simulink model "cooSim"  (R2018b)
settings: Solver=VariableStepAuto  StartTime=0.0  StopTime=Time(end)  RelTol=1e-3
values from neighbouring files (symbols this model uses):
  A = [lang.velocity.x(i) lang.velocity.y(i)]'    [DataTreatment.m]    (also in coo.m = [)
  B = [ ... (first row only)    [coo.m]
  C = (R^-1)*A    [DataTreatment.m]    (also in coo.m = [)
  c = rms(sqrt(a.^2+b.^2))    [coo.m]
  D = [ ... (first row only)    [coo.m]
  iz = 4.192e3    (= 4192)    [coo.m]
  Ki = lqi(Gpss,Q,R)    [coo.m]
  lf = cog_x*L    (= 0.70125)    [coo.m]
  lr = (1-cog_x)*L    (= 2.10375)    [coo.m]
  m = m(trimstart:end-trimend,:)    [DataTreatment.m]    (also in coo.m = mean([1684 1774]))
  swaThreshold = 5    [coo.m]
  TH = 9999    [coo.m]
  vxThreshold = 1    [coo.m]
  yawThreshold = 0.1    [coo.m]
undefined symbols (not defined in the file or in its folder): K, Vehicle
libraries: simulink_extras x1
settings Model: Creator=carl  LastModifiedBy=carl

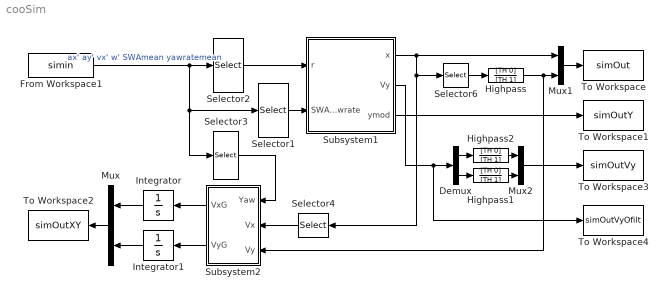
== system cooSim ==
  Demux : Demux  Outputs=2
  From Workspace1 : FromWorkspace  VariableName=simin  SampleTime=0
  Highpass : TransferFcn  Numerator=[TH 0]  Denominator=[TH 1]
  Highpass1 : TransferFcn  Numerator=[TH 0]  Denominator=[TH 1]
  Highpass2 : TransferFcn  Numerator=[TH 0]  Denominator=[TH 1]
  Integrator : Integrator
  Integrator1 : Integrator
  Mux : Mux  Inputs=2
  Mux1 : Mux  Inputs=2
  Mux2 : Mux  Inputs=2
  Selector1 : Selector  InputPortWidth=7  IndexOptions=Index vector (dialog)  Indices=[3,6,7]  OutputSizes=1
  Selector2 : Selector  InputPortWidth=7  IndexOptions=Index vector (dialog)  Indices=[1 2 3 4]  OutputSizes=1
  Selector3 : Selector  InputPortWidth=7  IndexOptions=Index vector (dialog)  Indices=[5]  OutputSizes=1
  Selector4 : Selector  InputPortWidth=3  IndexOptions=Index vector (dialog)  Indices=[1]  OutputSizes=1
  Selector6 : Selector  InputPortWidth=3  IndexOptions=Index vector (dialog)  Indices=[2]  OutputSizes=1
  Subsystem1 : Subsystem
  Subsystem2 : Subsystem
  To Workspace : ToWorkspace  VariableName=simOut  SaveFormat=Timeseries  SampleTime=-1
  To Workspace1 : ToWorkspace  VariableName=simOutY  SaveFormat=Timeseries  SampleTime=-1
  To Workspace2 : ToWorkspace  VariableName=simOutXY  SaveFormat=Timeseries  SampleTime=-1
  To Workspace3 : ToWorkspace  VariableName=simOutVy  SaveFormat=Timeseries  SampleTime=-1
  To Workspace4 : ToWorkspace  VariableName=simOutVyOfilt  SaveFormat=Timeseries  SampleTime=-1
  wires:
  From Workspace1/1 -> Selector1/1, Selector3/1, Selector2/1  "ax' ay' vx' w' SWAmean yawratemean"
  Subsystem1/1(x) -> Selector4/1, Selector6/1, Mux1/1
  Subsystem1/3(ymod) -> To Workspace1/1
  Subsystem2/1(VxG) -> Integrator/1
  Subsystem2/2(VyG) -> Integrator1/1
  Selector3/1 -> Subsystem2/1(Yaw)
  Integrator1/1 -> Mux/2
  Integrator/1 -> Mux/1
  Mux/1 -> To Workspace2/1
  Selector4/1 -> Subsystem2/2(Vx)
  Mux1/1 -> To Workspace/1
  Selector6/1 -> Highpass/1
  Subsystem1/2(Vy) -> To Workspace4/1, Demux/1
  Highpass1/1 -> Mux2/2
  Highpass2/1 -> Mux2/1
  Mux2/1 -> To Workspace3/1
  Demux/1 -> Highpass2/1
  Demux/2 -> Highpass1/1
  Selector2/1 -> Subsystem1/1(r)
  Selector1/1 -> Subsystem1/2(SWA yawrate)
  Highpass/1 -> Subsystem2/3(Vy), Mux1/2

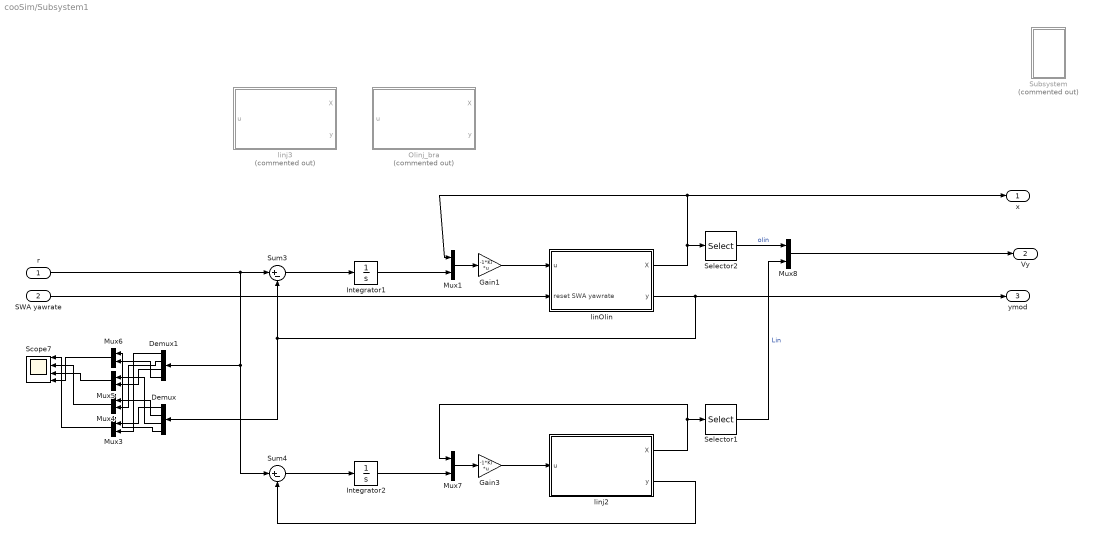
== system cooSim/Subsystem1 ==
  r : Inport
  SWA yawrate : Inport  Port=2
  Demux : Demux
  Demux1 : Demux
  Gain1 : Gain  Gain=-1*Ki  Multiplication=Matrix(K*u) (u vector)
  Gain3 : Gain  Gain=-1*Ki  Multiplication=Matrix(K*u) (u vector)
  Integrator1 : Integrator
  Integrator2 : Integrator
  Mux{1,3..8} (7 alike) : Mux  Inputs=2
  Olinj_bra : Subsystem  Commented=on
  Scope7 : Scope  NumInputPorts=4
  Selector1 : Selector  InputPortWidth=3  IndexOptions=Index vector (dialog)  Indices=2  OutputSizes=1
  Selector2 : Selector  InputPortWidth=3  IndexOptions=Index vector (dialog)  Indices=2  OutputSizes=1
  Subsystem : Subsystem  Commented=on
  Sum3 : Sum  Inputs=|+-
  Sum4 : Sum  Inputs=|+-
  linOlin : Subsystem
  linj2 : Subsystem
  linj3 : Subsystem  Commented=on
  x : Outport
  Vy : Outport  Port=2
  ymod : Outport  Port=3
  wires:
  Sum3/1 -> Integrator1/1
  Gain1/1 -> linOlin/1(u)
  linOlin/2(y) -> Demux/1, Sum3/2, ymod/1
  linOlin/1(X) -> x/1, Mux1/1, Selector2/1
  Mux1/1 -> Gain1/1
  Integrator1/1 -> Mux1/2
  r/1 -> Demux1/1, Sum4/1, Sum3/1
  Selector2/1 -> Mux8/1  "olin"
  Mux3/1 -> Scope7/1
  Mux4/1 -> Scope7/2
  Mux5/1 -> Scope7/3
  Mux6/1 -> Scope7/4
  Demux/1 -> Mux3/1
  Demux1/1 -> Mux3/2
  Demux/2 -> Mux4/1
  Demux1/2 -> Mux4/2
  Demux/3 -> Mux5/1
  Demux1/3 -> Mux5/2
  Demux/4 -> Mux6/1
  Demux1/4 -> Mux6/2
  Selector1/1 -> Mux8/2  "Lin"
  Integrator2/1 -> Mux7/2
  Mux7/1 -> Gain3/1
  linj2/1(X) -> Mux7/1, Selector1/1
  linj2/2(y) -> Sum4/2
  Gain3/1 -> linj2/1(u)
  Sum4/1 -> Integrator2/1
  Mux8/1 -> Vy/1
  SWA yawrate/1 -> linOlin/2(reset SWA yawrate)

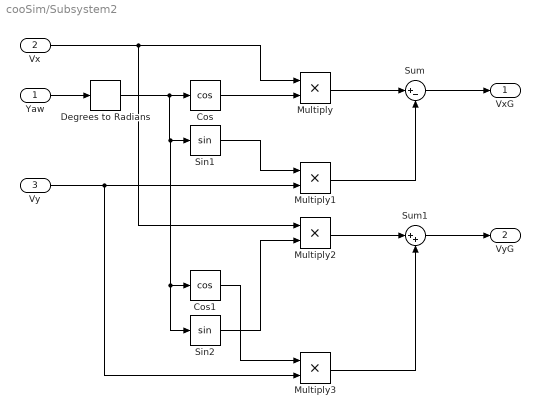
== system cooSim/Subsystem2 ==
  Yaw : Inport
  Vx : Inport  Port=2
  Vy : Inport  Port=3
  Cos : Trigonometry  Operator=cos
  Cos1 : Trigonometry  Operator=cos
  Degrees to Radians : simulink_extras/Transformations/Degrees to Radians
  Multiply{,1..3} (4 alike) : Product
  Sin1 : Trigonometry
  Sin2 : Trigonometry
  Sum : Sum  Inputs=|+-
  Sum1 : Sum  Inputs=|++
  VxG : Outport
  VyG : Outport  Port=2
  wires:
  Multiply/1 -> Sum/1
  Cos/1 -> Multiply/2
  Sin1/1 -> Multiply1/1
  Multiply1/1 -> Sum/2
  Sum/1 -> VxG/1
  Multiply2/1 -> Sum1/1
  Vx/1 -> Multiply2/1, Multiply/1
  Multiply3/1 -> Sum1/2
  Vy/1 -> Multiply1/2, Multiply3/2
  Sum1/1 -> VyG/1
  Sin2/1 -> Multiply2/2
  Cos1/1 -> Multiply3/1
  Yaw/1 -> Degrees to Radians/1
  Degrees to Radians/1 -> Sin2/1, Cos1/1, Sin1/1, Cos/1

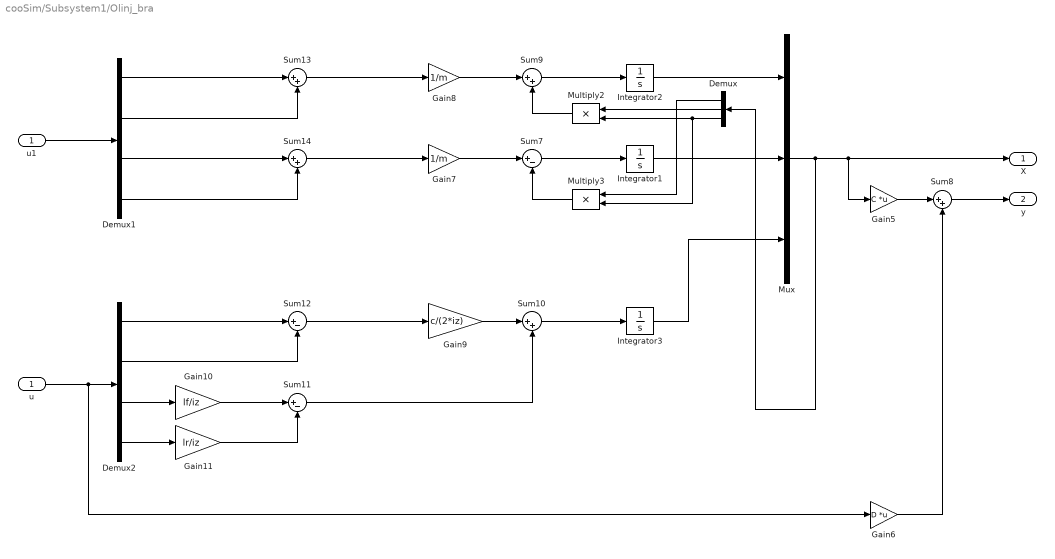
== system cooSim/Subsystem1/Olinj_bra ==
  u : Inport
  Demux : Demux  Outputs=3
  Demux1 : Demux
  Demux2 : Demux
  Gain10 : Gain  Gain=lf/iz
  Gain11 : Gain  Gain=lr/iz
  Gain5 : Gain  Gain=C  Multiplication=Matrix(K*u) (u vector)
  Gain6 : Gain  Gain=D  Multiplication=Matrix(K*u) (u vector)
  Gain7 : Gain  Gain=1/m
  Gain8 : Gain  Gain=1/m
  Gain9 : Gain  Gain=c/(2*iz)
  Integrator1 : Integrator
  Integrator2 : Integrator
  Integrator3 : Integrator
  Multiply2 : Product
  Multiply3 : Product
  Mux : Mux  Inputs=3
  Sum{8..10,13..14} (5 alike) : Sum  Inputs=|++
  Sum11 : Sum  Inputs=|+-
  Sum12 : Sum  Inputs=|+-
  Sum7 : Sum  Inputs=|+-
  u1 : InportShadow
  X : Outport
  y : Outport  Port=2
  wires:
  Gain5/1 -> Sum8/1
  Gain6/1 -> Sum8/2
  Sum8/1 -> y/1
  Gain7/1 -> Sum7/1
  Sum7/1 -> Integrator1/1
  Gain8/1 -> Sum9/1
  Sum9/1 -> Integrator2/1
  Multiply2/1 -> Sum9/2
  Multiply3/1 -> Sum7/2
  Sum10/1 -> Integrator3/1
  Gain9/1 -> Sum10/1
  Gain10/1 -> Sum11/1
  Gain11/1 -> Sum11/2
  u/1 -> Gain6/1, Demux2/1
  Demux2/1 -> Sum12/1
  Demux2/2 -> Sum12/2
  Sum12/1 -> Gain9/1
  Demux2/3 -> Gain10/1
  Demux2/4 -> Gain11/1
  Sum11/1 -> Sum10/2
  u1/1 -> Demux1/1
  Demux1/1 -> Sum13/1
  Demux1/2 -> Sum13/2
  Demux1/3 -> Sum14/1
  Demux1/4 -> Sum14/2
  Sum13/1 -> Gain8/1
  Sum14/1 -> Gain7/1
  Integrator3/1 -> Mux/3
  Integrator1/1 -> Mux/2
  Integrator2/1 -> Mux/1
  Demux/2 -> Multiply2/1
  Demux/1 -> Multiply3/1
  Demux/3 -> Multiply3/2, Multiply2/2
  Mux/1 -> X/1, Gain5/1, Demux/1

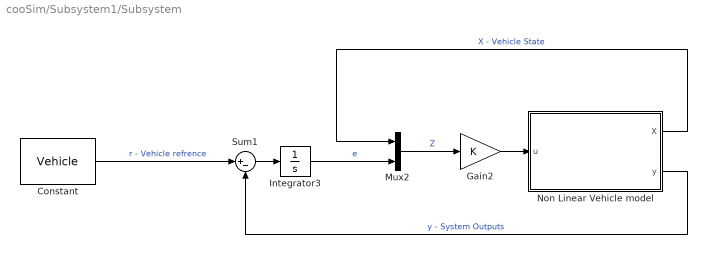
== system cooSim/Subsystem1/Subsystem ==
  Constant : Constant  Value=Vehicle
  Gain2 : Gain  Gain=K
  Integrator3 : Integrator
  Mux2 : Mux  Inputs=2
  Non Linear Vehicle model : Subsystem
  Sum1 : Sum  Inputs=|+-
  wires:
  Gain2/1 -> Non Linear Vehicle model/1(u)
  Sum1/1 -> Integrator3/1
  Constant/1 -> Sum1/1  "r - Vehicle refrence"
  Mux2/1 -> Gain2/1  "Z"
  Non Linear Vehicle model/1(X) -> Mux2/1  "X - Vehicle State"
  Non Linear Vehicle model/2(y) -> Sum1/2  "y - System Outputs"
  Integrator3/1 -> Mux2/2  "e"

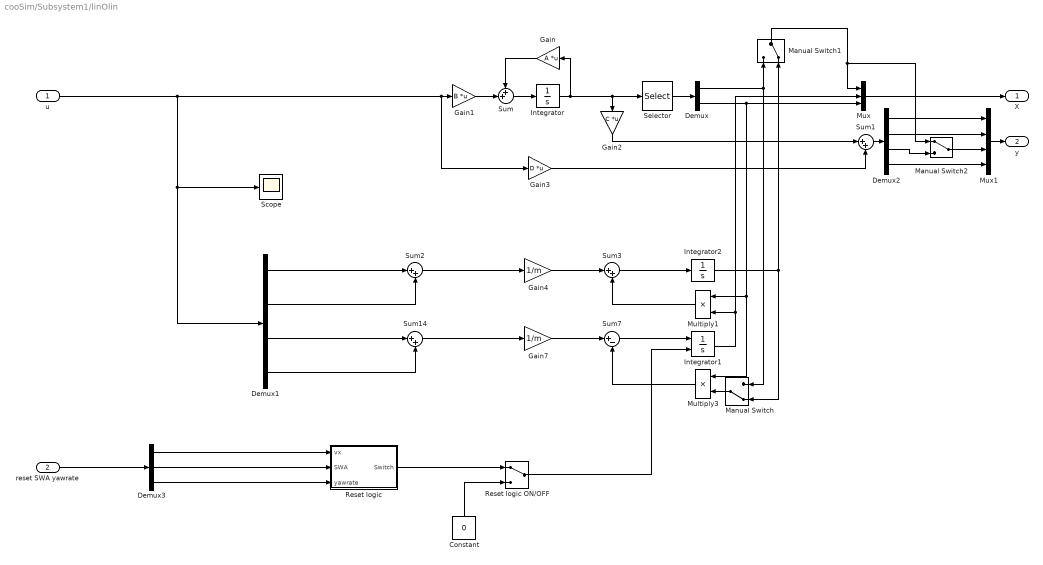
== system cooSim/Subsystem1/linOlin ==
  u : Inport
  reset SWA yawrate : Inport  Port=2
  Constant : Constant  Value=0
  Demux : Demux  Outputs=2
  Demux1 : Demux
  Demux2 : Demux
  Demux3 : Demux  Outputs=3
  Gain : Gain  Gain=A  Multiplication=Matrix(K*u) (u vector)
  Gain1 : Gain  Gain=B  Multiplication=Matrix(K*u) (u vector)
  Gain2 : Gain  Gain=C  Multiplication=Matrix(K*u) (u vector)
  Gain3 : Gain  Gain=D  Multiplication=Matrix(K*u) (u vector)
  Gain4 : Gain  Gain=1/m
  Gain7 : Gain  Gain=1/m
  Integrator : Integrator
  Integrator1 : Integrator  ExternalReset=rising
  Integrator2 : Integrator
  Manual Switch : ManualSwitch  CurrentSetting=0
  Manual Switch1 : ManualSwitch  CurrentSetting=0
  Manual Switch2 : ManualSwitch
  Multiply1 : Product
  Multiply3 : Product
  Mux : Mux  Inputs=3
  Mux1 : Mux
  Reset logic : Subsystem
  Reset logic ON/OFF : ManualSwitch
  Scope : Scope
  Selector : Selector  InputPortWidth=3  IndexOptions=Index vector (dialog)  Indices=[1 3]  OutputSizes=1
  Sum : Sum  Inputs=++|
  Sum{1..3,14} (4 alike) : Sum  Inputs=|++
  Sum7 : Sum  Inputs=|+-
  X : Outport
  y : Outport  Port=2
  wires:
  Sum1/1 -> Demux2/1
  Sum/1 -> Integrator/1
  Integrator/1 -> Gain2/1, Selector/1, Gain/1
  Gain/1 -> Sum/1
  Gain1/1 -> Sum/2
  Gain2/1 -> Sum1/1
  Gain3/1 -> Sum1/2
  Demux/1 -> Manual Switch/1, Manual Switch1/1
  Demux1/4 -> Sum14/2
  Sum7/1 -> Integrator1/1
  Multiply3/1 -> Sum7/2
  Demux1/3 -> Sum14/1
  Sum14/1 -> Gain7/1
  Integrator1/1 -> Multiply1/2, Mux/2
  u/1 -> Gain3/1, Gain1/1, Demux1/1, Scope/1
  Gain7/1 -> Sum7/1
  Demux/2 -> Mux/3, Multiply1/1, Multiply3/1
  Selector/1 -> Demux/1
  Mux/1 -> X/1
  Gain4/1 -> Sum3/1
  Sum2/1 -> Gain4/1
  Demux1/1 -> Sum2/1
  Multiply1/1 -> Sum3/2
  Sum3/1 -> Integrator2/1
  Demux1/2 -> Sum2/2
  Integrator2/1 -> Manual Switch1/2, Manual Switch/2
  Manual Switch/1 -> Multiply3/2
  Manual Switch1/1 -> Manual Switch2/1, Mux/1
  Mux1/1 -> y/1
  Demux2/1 -> Mux1/1
  Demux2/2 -> Mux1/2
  Demux2/4 -> Mux1/4
  Demux2/3 -> Manual Switch2/2
  Manual Switch2/1 -> Mux1/3
  Reset logic/1(Switch) -> Reset logic ON/OFF/1
  reset SWA yawrate/1 -> Demux3/1
  Demux3/1 -> Reset logic/1(vx)
  Demux3/2 -> Reset logic/2(SWA)
  Demux3/3 -> Reset logic/3(yawrate)
  Reset logic ON/OFF/1 -> Integrator1/2
  Constant/1 -> Reset logic ON/OFF/2

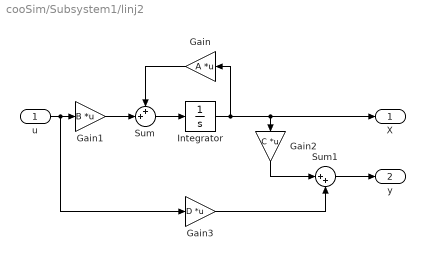
== system cooSim/Subsystem1/linj2 ==
  u : Inport
  Gain : Gain  Gain=A  Multiplication=Matrix(K*u) (u vector)
  Gain1 : Gain  Gain=B  Multiplication=Matrix(K*u) (u vector)
  Gain2 : Gain  Gain=C  Multiplication=Matrix(K*u) (u vector)
  Gain3 : Gain  Gain=D  Multiplication=Matrix(K*u) (u vector)
  Integrator : Integrator
  Sum : Sum  Inputs=++|
  Sum1 : Sum  Inputs=|++
  X : Outport
  y : Outport  Port=2
  wires:
  Sum1/1 -> y/1
  Sum/1 -> Integrator/1
  Integrator/1 -> X/1, Gain2/1, Gain/1
  Gain/1 -> Sum/1
  u/1 -> Gain3/1, Gain1/1
  Gain1/1 -> Sum/2
  Gain2/1 -> Sum1/1
  Gain3/1 -> Sum1/2

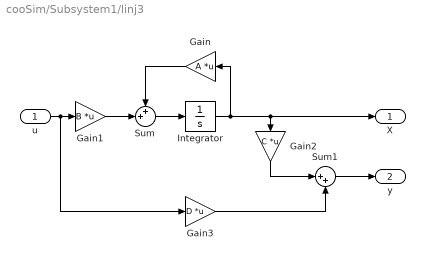
== system cooSim/Subsystem1/linj3 ==
  u : Inport
  Gain : Gain  Gain=A  Multiplication=Matrix(K*u) (u vector)
  Gain1 : Gain  Gain=B  Multiplication=Matrix(K*u) (u vector)
  Gain2 : Gain  Gain=C  Multiplication=Matrix(K*u) (u vector)
  Gain3 : Gain  Gain=D  Multiplication=Matrix(K*u) (u vector)
  Integrator : Integrator
  Sum : Sum  Inputs=++|
  Sum1 : Sum  Inputs=|++
  X : Outport
  y : Outport  Port=2
  wires:
  Gain3/1 -> Sum1/2
  Gain2/1 -> Sum1/1
  Gain1/1 -> Sum/2
  u/1 -> Gain1/1, Gain3/1
  Gain/1 -> Sum/1
  Integrator/1 -> Gain/1, Gain2/1, X/1
  Sum/1 -> Integrator/1
  Sum1/1 -> y/1

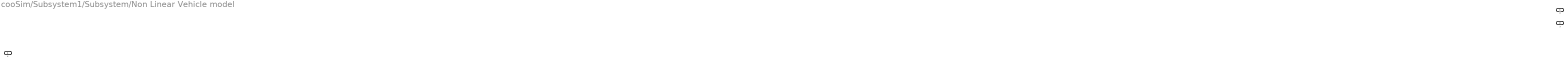
== system cooSim/Subsystem1/Subsystem/Non Linear Vehicle model ==
  u : Inport
  X : Outport
  y : Outport  Port=2

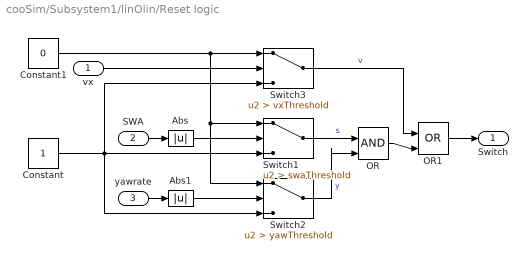
== system cooSim/Subsystem1/linOlin/Reset logic ==
  vx : Inport
  SWA : Inport  Port=2
  yawrate : Inport  Port=3
  Abs : Abs
  Abs1 : Abs
  Constant : Constant
  Constant1 : Constant  Value=0
  OR : Logic  IconShape=distinctive  AllPortsSameDT=off  OutDataTypeStr=boolean
  OR1 : Logic  Operator=OR  IconShape=distinctive  AllPortsSameDT=off  OutDataTypeStr=boolean
  Switch1 : Switch  Criteria=u2 > Threshold  Threshold=swaThreshold
  Switch2 : Switch  Criteria=u2 > Threshold  Threshold=yawThreshold
  Switch3 : Switch  Criteria=u2 > Threshold  Threshold=vxThreshold
  Switch : Outport
  wires:
  SWA/1 -> Abs/1
  yawrate/1 -> Abs1/1
  Constant/1 -> Switch1/3, Switch3/3, Switch2/3
  Constant1/1 -> Switch1/1, Switch2/1, Switch3/1
  Switch1/1 -> OR/1  "s"
  Switch2/1 -> OR/2  "y"
  OR/1 -> OR1/2
  Abs/1 -> Switch1/2
  Abs1/1 -> Switch2/2
  vx/1 -> Switch3/2
  Switch3/1 -> OR1/1  "v"
  OR1/1 -> Switch/1
